simulink model "SatSim_ARES_prototype"  (R2022b)
settings: Solver=VariableStepAuto  StartTime=0.0  StopTime=100  RelTol=1e-3
values from neighbouring files (symbols this model uses):
  BC = m/A/Cd    (= 136.363636364)    [ARES.m]    (also in control_before_MPC.m = 122; reference_signal_291123.m = 121.212121212; validation.m)
  Cd = 2.2    [ARES.m]    (also in control_before_MPC.m; control_script_291123.m; reference_signal_291123.m; validation.m)
  CL = Cd*E    (= 0)    [ARES.m]    (also in control_before_MPC.m; control_script_291123.m; reference_signal_291123.m; validation.m)
  F107_avg = 90.85    [ARES.m]    (also in control_before_MPC.m; control_script_291123.m; reference_signal_291123.m; validation.m)
  F107_day = 86.0    (= 86)    [ARES.m]    (also in control_before_MPC.m; control_script_291123.m; reference_signal_291123.m; validation.m)
  jdate = jdate+ndays1    [ARES.m]    (also in control_before_MPC.m; control_script_291123.m; reference_signal_291123.m; validation.m)
  Kp = 1    [ARES.m]    (also in control_before_MPC.m; control_script_291123.m; reference_signal_291123.m; validation.m)
  mi = 398600.44    [ARES.m]    (also in control_before_MPC.m; control_script_291123.m; reference_signal_291123.m; validation.m)
  r_a = alt_0+Re    (= 6771.0088)    [ARES.m]    (also in control_before_MPC.m = 6571.0088; control_script_291123.m = 6571.0088; reference_signal_291123.m = 6571.0088; validation.m)
  Re = Re*1000    (= 6371008.8)    [ARES.m]    (also in control_before_MPC.m; control_script_291123.m; reference_signal_291123.m; trajectory_solver.m = 6378000)
  stop_h = 0    [ARES.m]    (also in control_before_MPC.m; control_script_291123.m; reference_signal_291123.m; validation.m)
libraries: simulink x2
settings Model: PauseTimes=0  Creator=zhanghanwen  LastModifiedBy=zhanghanwen

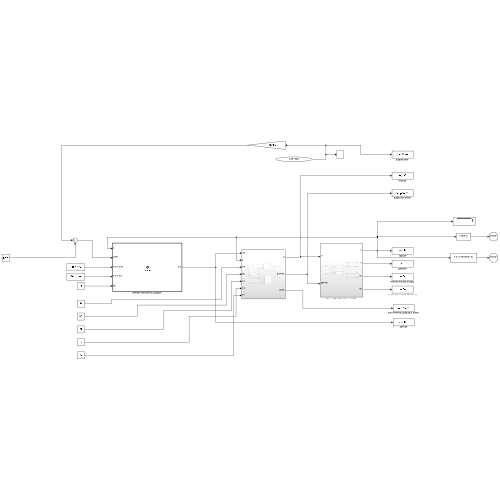
[thumbnail: Simulink's stored preview of the top-level diagram]
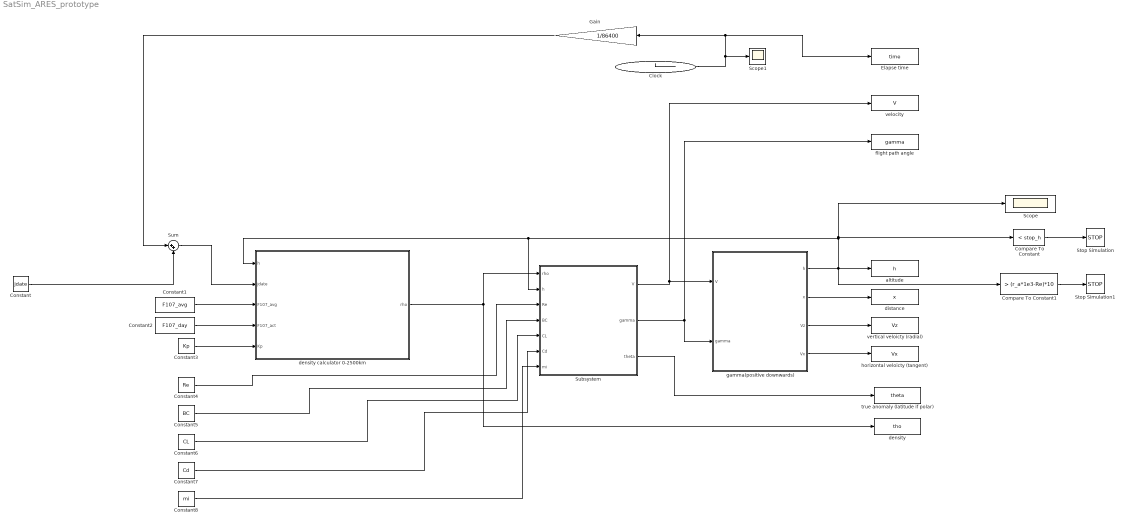
== system SatSim_ARES_prototype ==
  Clock : Clock
  Compare To Constant : simulink/Logic and Bit Operations/Compare To Constant  relop=<  const=stop_h  OutDataTypeStr=boolean
  Compare To Constant1 : simulink/Logic and Bit Operations/Compare To Constant  relop=>  const=(r_a*1e3-Re)*10  OutDataTypeStr=boolean
  Constant : Constant  Value=jdate
  Constant1 : Constant  Value=F107_avg
  Constant2 : Constant  Value=F107_day
  Constant3 : Constant  Value=Kp
  Constant4 : Constant  Value=Re
  Constant5 : Constant  Value=BC
  Constant6 : Constant  Value=CL
  Constant7 : Constant  Value=Cd
  Constant8 : Constant  Value=mi
  Elapse time : ToWorkspace  VariableName=time  SampleTime=-1
      settings: Save2DSignal=2-D array (concatenate along first dimension)
  Gain : Gain  Gain=1/86400
  Scope : Scope
  Scope1 : Scope
  Stop Simulation : Stop
  Stop Simulation1 : Stop
  Subsystem : Subsystem
  Sum : Sum  Inputs=|++
  altitude : ToWorkspace  VariableName=h  SampleTime=-1
      settings: Save2DSignal=2-D array (concatenate along first dimension)
  density : ToWorkspace  VariableName=tho  SampleTime=-1
      settings: Save2DSignal=2-D array (concatenate along first dimension)
  density calculator 0-2500km : MATLAB Function  TreatAsAtomicUnit=on
  distance : ToWorkspace  VariableName=x  SampleTime=-1
      settings: Save2DSignal=2-D array (concatenate along first dimension)
  flight path angle : ToWorkspace  VariableName=gamma  SampleTime=-1
      settings: Save2DSignal=2-D array (concatenate along first dimension)
  gamma(positive downwards) : Subsystem
  horizontal veloicty (tangent) : ToWorkspace  VariableName=Vx  SampleTime=-1
      settings: Save2DSignal=2-D array (concatenate along first dimension)
  true anomaly (latitude if polar) : ToWorkspace  VariableName=theta  SampleTime=-1
      settings: Save2DSignal=2-D array (concatenate along first dimension)
  velocity : ToWorkspace  VariableName=V  SampleTime=-1
      settings: Save2DSignal=2-D array (concatenate along first dimension)
  vertical veloicty (radial) : ToWorkspace  VariableName=Vz  SampleTime=-1
      settings: Save2DSignal=2-D array (concatenate along first dimension)
  wires:
  Constant1/1 -> density calculator 0-2500km/3(F107_avg)
  Constant3/1 -> density calculator 0-2500km/5(Kp)
  Constant2/1 -> density calculator 0-2500km/4(F107_act)
  Constant/1 -> Sum/2
  density calculator 0-2500km/1(rho) -> density/1, Subsystem/1(rho)
  Subsystem/1(V) -> velocity/1, gamma(positive downwards)/1(V)
  Subsystem/2(gamma) -> flight path angle/1, gamma(positive downwards)/2(gamma)
  gamma(positive downwards)/2(x) -> distance/1
  gamma(positive downwards)/3(Vz) -> vertical veloicty (radial)/1
  gamma(positive downwards)/4(Vx) -> horizontal veloicty (tangent)/1
  gamma(positive downwards)/1(h) -> Scope/1, Compare To Constant/1, density calculator 0-2500km/1(h), Subsystem/2(h), altitude/1, Compare To Constant1/1
  Compare To Constant1/1 -> Stop Simulation1/1
  Compare To Constant/1 -> Stop Simulation/1
  Subsystem/3(theta) -> true anomaly (latitude if polar)/1
  Gain/1 -> Sum/1
  Sum/1 -> density calculator 0-2500km/2(jdate)
  Constant6/1 -> Subsystem/5(CL)
  Constant5/1 -> Subsystem/4(BC)
  Constant7/1 -> Subsystem/6(Cd)
  Constant4/1 -> Subsystem/3(Re)
  Constant8/1 -> Subsystem/7(mi)
  Clock/1 -> Elapse time/1, Gain/1, Scope1/1

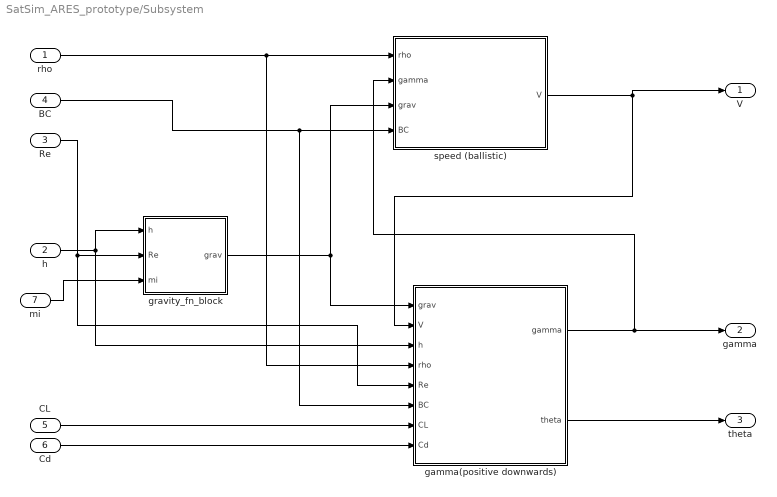
== system SatSim_ARES_prototype/Subsystem ==
  rho : Inport
  h : Inport  Port=2
  Re : Inport  Port=3
  BC : Inport  Port=4
  CL : Inport  Port=5
  Cd : Inport  Port=6
  mi : Inport  Port=7
  gamma(positive downwards) : Subsystem
  gravity_fn_block : MATLAB Function  TreatAsAtomicUnit=on
  speed (ballistic) : Subsystem
  V : Outport
  gamma : Outport  Port=2
  theta : Outport  Port=3
  wires:
  rho/1 -> gamma(positive downwards)/4(rho), speed (ballistic)/1(rho)
  gravity_fn_block/1(grav) -> speed (ballistic)/3(grav), gamma(positive downwards)/1(grav)
  h/1 -> gamma(positive downwards)/3(h), gravity_fn_block/1(h)
  gamma(positive downwards)/1(gamma) -> speed (ballistic)/2(gamma), gamma/1
  gamma(positive downwards)/2(theta) -> theta/1
  speed (ballistic)/1(V) -> V/1, gamma(positive downwards)/2(V)
  Re/1 -> gamma(positive downwards)/5(Re), gravity_fn_block/2(Re)
  BC/1 -> gamma(positive downwards)/6(BC), speed (ballistic)/4(BC)
  CL/1 -> gamma(positive downwards)/7(CL)
  Cd/1 -> gamma(positive downwards)/8(Cd)
  mi/1 -> gravity_fn_block/3(mi)

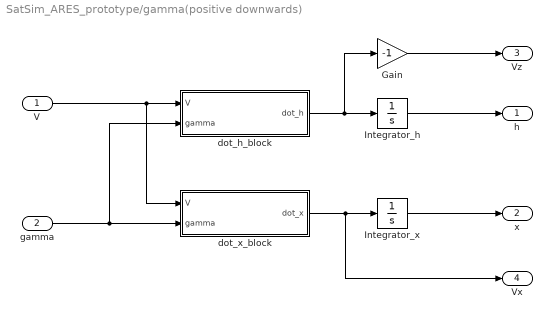
== system SatSim_ARES_prototype/gamma(positive downwards) ==
  V : Inport
  gamma : Inport  Port=2
  Gain : Gain  Gain=-1
  Integrator_h : Integrator
  Integrator_x : Integrator
  dot_h_block : MATLAB Function  TreatAsAtomicUnit=on
  dot_x_block : MATLAB Function  TreatAsAtomicUnit=on
  h : Outport
  x : Outport  Port=2
  Vz : Outport  Port=3
  Vx : Outport  Port=4
  wires:
  V/1 -> dot_x_block/1(V), dot_h_block/1(V)
  gamma/1 -> dot_x_block/2(gamma), dot_h_block/2(gamma)
  Integrator_h/1 -> h/1
  dot_h_block/1(dot_h) -> Gain/1, Integrator_h/1
  Integrator_x/1 -> x/1
  dot_x_block/1(dot_x) -> Vx/1, Integrator_x/1
  Gain/1 -> Vz/1

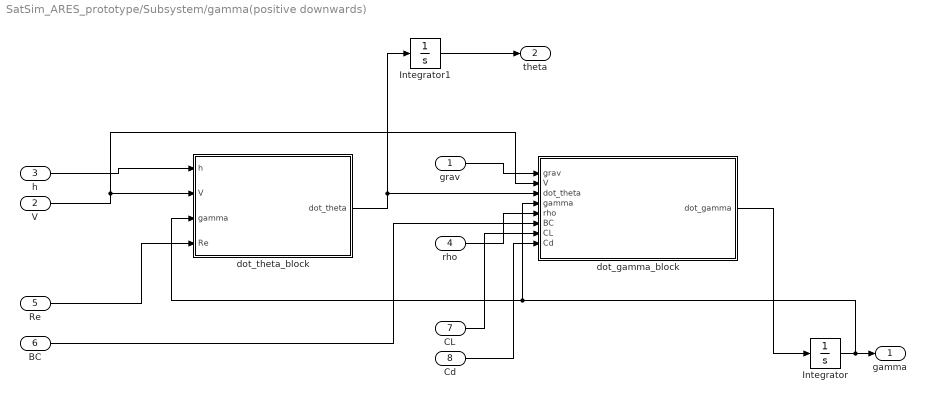
== system SatSim_ARES_prototype/Subsystem/gamma(positive downwards) ==
  grav : Inport
  V : Inport  Port=2
  h : Inport  Port=3
  rho : Inport  Port=4
  Re : Inport  Port=5
  BC : Inport  Port=6
  CL : Inport  Port=7
  Cd : Inport  Port=8
  Integrator : Integrator
  Integrator1 : Integrator
  dot_gamma_block : MATLAB Function  TreatAsAtomicUnit=on
  dot_theta_block : MATLAB Function  TreatAsAtomicUnit=on
  gamma : Outport
  theta : Outport  Port=2
  wires:
  grav/1 -> dot_gamma_block/1(grav)
  dot_gamma_block/1(dot_gamma) -> Integrator/1
  dot_theta_block/1(dot_theta) -> Integrator1/1, dot_gamma_block/3(dot_theta)
  rho/1 -> dot_gamma_block/5(rho)
  h/1 -> dot_theta_block/1(h)
  V/1 -> dot_gamma_block/2(V), dot_theta_block/2(V)
  Integrator1/1 -> theta/1
  Integrator/1 -> dot_theta_block/3(gamma), dot_gamma_block/4(gamma), gamma/1
  Re/1 -> dot_theta_block/4(Re)
  BC/1 -> dot_gamma_block/6(BC)
  CL/1 -> dot_gamma_block/7(CL)
  Cd/1 -> dot_gamma_block/8(Cd)

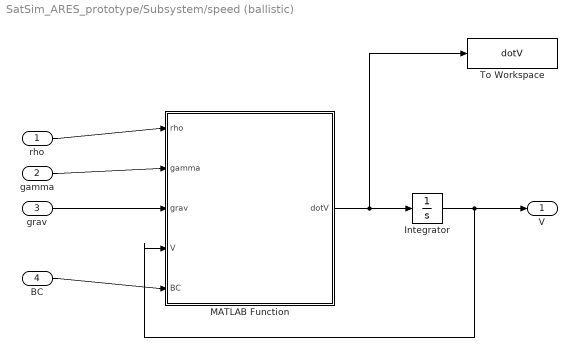
== system SatSim_ARES_prototype/Subsystem/speed (ballistic) ==
  rho : Inport
  gamma : Inport  Port=2
  grav : Inport  Port=3
  BC : Inport  Port=4
  Integrator : Integrator
  MATLAB Function : MATLAB Function  TreatAsAtomicUnit=on
  To Workspace : ToWorkspace  VariableName=dotV  SaveFormat=Timeseries  SampleTime=-1
  V : Outport
  wires:
  Integrator/1 -> MATLAB Function/4(V), V/1
  grav/1 -> MATLAB Function/3(grav)
  gamma/1 -> MATLAB Function/2(gamma)
  rho/1 -> MATLAB Function/1(rho)
  MATLAB Function/1(dotV) -> To Workspace/1, Integrator/1
  BC/1 -> MATLAB Function/5(BC)

== matlab function SatSim_ARES_prototype/Subsystem/gravity_fn_block ==
  data: h input; grav output; Re input; mi input
function grav = gravity(h,Re,mi)

grav = mi*1e9 / (Re+h)^2;
end

== matlab function SatSim_ARES_prototype/density calculator 0-2500km ==
  data: h input; jdate input; F107_avg input; rho output; F107_act input; Kp input
%This function combines Jacchia J71 and Exponential Atmosphere for %calculating density in the band [0;2500] km
%A transition function should be introduced to avoid discontinuities
function rho = unirho(h,jdate,F107_avg,F107_act,Kp) 
     h=h/1000; %conversion [m] to [km]
    rho=0;
    %from 0 to 100 km of altitude use Exponential Atmosphere
    if h<100 && h>=0
        rho=expAtm(h);
    end
    %from 100 to 2500 km of altitude use Jacchia J71
    if h>=100 && h<=2500 
       rho=J71_density_simulink(h,jdate,F107_avg,F107_act,Kp);
    end
    %A warning is printed if a negative altitude is predicted by %the simulation (due to Simulink discrete stopping criterion)
    if h<0
       fprintf('Warning: mismatched density, altitude: %3.2e km',h) 
       rho=1.225;
    end
end



%This function computes the density using Jacchia J71 model
%rho=J71_density_simulink(H,jdate,F107_avg,F107_act,Kp)
%input: height [90-2500 km], julian date, F10.7 3-monthly average, F10.7
%three hourly average, Kp planetary index
%output: density value
%Reference: Satellite Orbits, section 3.5.3
function rho=J71_density_simulink(H,jdate,F107_avg,F107_act,Kp)

    %% Exosperic Temperature 
    T_c = 379.0+3.24*F107_avg+1.3*(F107_act-F107_avg);
    % Geographic corrections
    % The actual exospheric temperature depends on the local hour angle
    % of the Sun with respect to the satellite.
    % It also depends, however, on the declination of the Sun and the
    % geographic latitude of the satellite.
    % The actual exospheric temperature T1 with the diurnal variations
    % included can be computed from a more compliated formula available
    % in the referenced book.
    % Geomagnetic corrections
    % using the three-hourly planetary geomagnetic index Kp for a time
    % 6.7 hours earlier than the time under consideration
    f = 0.5*(tanh(0.04*(H-350)+1));
    dT_infH = 28.0*Kp+0.03*exp(Kp);
    dT_infL = 14.0*Kp+0.02*exp(Kp);
    dT_gm = f*dT_infH+(1-f)*dT_infL;
    %transition function
    %H>350km
    %H<350km
    T_e = T_c+dT_gm;   %geomagnetic corrected exospheric temperature
    
    %% Standard Density 
    %Use bi-polynomial fit from Gill (1996)
    coeff=getCoeff(H,T_e); %coefficient matrix
    logRho=0;
    for i=0:5
        for j=0:4
            logRho = logRho + coeff(i+1,j+1)*((H/1000)^i)*((T_e/1000)^j);
        end 
    end

    %% Corrections 
    %Correction due to semi-annual density variation in thermosphere
    Phi=(jdate - 2400000.5 -36204)/365.2422; %number of tropical years since Jan1, 1958
    
    tauSA=Phi + 0.09544*((0.5+0.5*sin(2*pi*Phi+6.035))^1.65 - 0.5);
    fZ=(5.876e-7*H^2.331 + 0.06328)*exp(H*-2.868e-3);
    gt=0.02835 + 0.3817*(1+0.4671*sin(2*pi*tauSA+4.137))*sin(4*pi*tauSA+4.259);
    logRhoSA=fZ*gt;
    %Correction due to geomagnetic activities
     if H<350
            logRhoGM = (0.012*Kp + 1.2e-5*exp(Kp))*(1-f);%Transition function from temp calc
     else
        logRhoGM=0;
     end
    %Seasonal-latitude correction
    %logRhoSL=0.014*(Z-90).*exp(-0.0013*(Z-90).^2)*sin(1*pi*Phi -1.72)*sin(lat)^3/abs(sin(lat));
    logRho=logRho+logRhoGM+logRhoSA;
    rho=10^logRho;
end

%This function calculates density through an exponential model
%rho=expAtm(H)
%H is the geopotential height in km
%rho is the density in kg/m^3
%rho0,h0,SH are updated each 10 km (source: Wertz, 1978)
function rho=expAtm(H)
[rho0,h0,SH]=getSH(H);
rho=rho0*exp(-(H-h0)/SH);   %kg/m^3
end

function c=getCoeff(Z,T)
    %Retrieve coefficients for bi-polynomial fit taken from Tables 3.9 and 3.10
    %of Satellite Orbits. These numbers were entered manually and may include
    %some typing errors. This should be replaced by the process described in
    %E. Gill, "Smooth Bi-Polynomial Interpolation of Jacchia 1971 Atmospheric
    %Densities For Efficient Satellite Drag Computation," DLR-GSOC IB 96-1,
    %German Aerospace Center (DLR), 1996
    %This paper is unavailable at this time.
    if Z<90 || Z>2500
        error('Z must be in range 90km < Z < 2500km')
    end
    if T<500 || T>1900
        error('T must be in range 500K < T < 1900K')
    end
    if T<850
        if Z<1000
            if Z<500
                if Z<180
                    c=[-0.3520856e2  0.3912622e1 -0.8649259e2  0.1504119e3 -0.7109428e2 ...
                        0.1129210e4  0.1198158e4  0.8633794e3 -0.3577091e4 -0.1970558e4 ...
                       -0.1527475e5 -0.3558481e5  0.1899243e5  0.2508241e5 -0.1968253e5 ...
                        0.9302042e5  0.3646554e6 -0.3290364e6 -0.1209631e5 0.8438137e5...
                       -0.2734394e6 -0.1576097e7  0.1685831e7 -0.4282943e6 -0.1345593e6...
                        0.3149696e6  0.2487723e7 -0.2899124e7  0.1111904e7 0.3294095e4];
                else
                    c=[ 0.2311910e2  0.1355298e3 -0.8424310e3  0.1287331e4 -0.6181209e3...
                       -0.1057776e4  0.6087973e3  0.8690566e4 -0.1715922e5 0.9052671e4...
                        0.1177230e5 -0.3164132e5 -0.1076323e4  0.6302629e5 -0.4312459e5...
                       -0.5827663e5  0.2188167e6 -0.2422912e6  0.2461286e5 0.6044096e5...
                        0.1254589e6 -0.5434710e6  0.8123016e6 -0.4490438e6 0.5007458e5...
                       -0.9452922e5  0.4408026e6 -0.7379410e6  0.5095273e6 -0.1154192e6];
                end
            else
                c=[-0.1815722e4  0.9792972e4 -0.1831374e5  0.1385255e5 -0.3451234e4...
                    0.9851221e4 -0.5397525e5  0.9993169e5 -0.7259456e5 0.1622553e5...
                   -0.1822932e5  0.1002430e6 -0.1784481e6  0.1145178e6 -0.1641934e5...
                    0.1298113e5 -0.7113430e5  0.1106375e6 -0.3825777e5 -0.1666915e5...
                   -0.1533510e4  0.7815537e4  0.7037562e4 -0.4674636e5 0.3516946e5...
                   -0.1263680e4  0.7265792e4 -0.2092909e5  0.2936094e5 -0.1491676e5];
            end
        else
            c=[ 0.3548698e3 -0.2508685e4  0.6252742e4 -0.6755376e4  0.2675763e4...
               -0.5370852e3  0.4182586e4 -0.1151114e5  0.1338915e5 -0.5610580e4...
               -0.2349586e2 -0.8941841e3  0.4417927e4 -0.6732817e4  0.3312608e4...
                0.3407073e3 -0.1531588e4  0.2179045e4 -0.8841341e3 -0.1369769e3...
               -0.1698470e3  0.8985697e3 -0.1704797e4  0.1363098e4 -0.3812417e3...
                0.2494943e2 -0.1389618e3  0.2820058e3 -0.2472862e3  0.7896439e2];
        end
    else 
        if Z<1000
            if Z<500
                if Z<180
                     c=[-0.5335412e2  0.2900557e2 -0.2046439e2  0.7977149e1 -0.1335853e1...
                         0.1977533e4 -0.7091478e3  0.4398538e3 -0.1568720e3 0.2615466e2...
                         -0.2993620e5  0.5187286e4 -0.1989795e4  0.3643166e3 -0.5700669e2...
                         0.2112068e6 -0.4483029e4 -0.1349971e5  0.9510012e4 -0.1653725e4...
                         -0.7209722e6 -0.7684101e5  0.1256236e6 -0.6805699e5 0.1181257e5...
                         0.9625966e6  0.2123127e6 -0.2622793e6  0.1337130e6 -0.2329995e5];
                else
                    c=[ 0.4041761e2 -0.1305719e3  0.1466809e3 -0.7120296e2 0.1269605e2...
                       -0.8127720e3  0.2273565e4 -0.2577261e4  0.1259045e4 -0.2254978e3...
                        0.5130043e4 -0.1501308e5  0.1717142e5 -0.8441698e4 0.1518796e4...
                       -0.1600170e5  0.4770469e5 -0.5473492e5  0.2699668e5 -0.4870306e4...
                        0.2384718e5 -0.7199064e5  0.8284653e5 -0.4098358e5 0.7411926e4...
                       -0.1363104e5  0.4153499e5 -0.4793581e5  0.2377854e5 -0.4310233e4];
                end
            else
                c=[-0.4021335e2 -0.1326983e3  0.3778864e3 -0.2808660e3 0.6513531e2...
                    0.4255789e3  0.3528126e3 -0.2077888e4  0.1726543e4 -0.4191477e3...
                   -0.1821662e4  0.7905357e3  0.3934271e4 -0.3969334e4 0.1027991e4...
                    0.3070231e4 -0.2941540e4 -0.3276639e4  0.4420217e4 -0.1230778e4...
                   -0.2196848e4  0.2585118e4  0.1382776e4 -0.2533006e4 0.7451387e3...
                    0.5494959e3 -0.6604225e3 -0.3328077e3  0.6335703e3 -0.1879812e3];
            end
        else 
            c=[ 0.1281061e2 -0.3389179e3  0.6861935e3 -0.4667627e3  0.1029662e3...
                0.2024251e3  0.1668302e3 -0.1147876e4  0.9918940e3 -0.2430215e3...
               -0.5750743e3  0.8259823e3  0.2329832e3 -0.6503359e3  0.1997989e3...
                0.5106207e3 -0.1032012e4  0.4851874e3  0.8214097e2 -0.6527048e2...
               -0.1898953e3  0.4347501e3 -0.2986011e3  0.5423180e2  0.5039459e1...
                0.2569577e2 -0.6282710e2  0.4971077e2 -0.1404385e2  0.8450500e0];
        end
    end
end


%[rho0,h0,SH]=getSH(H) this function gives coefficient for an exponential
% atmosphere model
%works below 100 km
function [rho0,h0,SH]=getSH(H)
    %input data from table 8-4 of Fundamentals of Astrodynamics, D.A. Vallado
    h0=[0,25,30,40,50,60,70,80,90];
    rho0=[1.225,3.899e-2,1.774e-2,3.972e-3,1.057e-3,3.206e-4,8.770e-5,1.905e-5,3.396e-6];
    SH=[7.249,6.349,6.682,7.554,8.382,7.714,6.549,5.799,5.382];
    n=fix(H/10);
    if H>100 || H<0
        error('H must be in the range 0km < H < 100 km; current value H=%.2fkm\n',H) 
    end
    if H<30 
        n=2;
        if H<25 
            n=1;
        end 
    end
    if H==100
        n=9;
    end
    h0=h0(n);
    rho0=rho0(n);
    SH=SH(n);
end

== matlab function SatSim_ARES_prototype/Subsystem/speed (ballistic)/MATLAB Function ==
  data: rho input; dotV output; gamma input; grav input; V input; BC input
function dotV = dvdt(rho,gamma,grav,V,BC)
dotV = -0.5*rho*V^2/BC + grav*sin(gamma);
end

== matlab function SatSim_ARES_prototype/Subsystem/gamma(positive downwards)/dot_theta_block ==
  data: h input; dot_theta output; V input; gamma input; Re input
function dot_theta = dthetadt(h,V,gamma,Re)

dot_theta = V*cos(gamma)/(Re+h); 

end

== matlab function SatSim_ARES_prototype/Subsystem/gamma(positive downwards)/dot_gamma_block ==
  data: grav input; dot_gamma output; V input; dot_theta input; gamma input; rho input; BC input; CL input; Cd input
function dot_gamma = dgammadt(grav,V,dot_theta,gamma,rho,BC,CL,Cd)
dot_gamma = grav / V * cos(gamma) -dot_theta- 0.5 * rho/BC * CL / Cd*V; 
end

== matlab function SatSim_ARES_prototype/gamma(positive downwards)/dot_h_block ==
  data: V input; dot_h output; gamma input
function dot_h = dhdt(V,gamma)
dot_h = -V*sin(gamma);
end

== matlab function SatSim_ARES_prototype/gamma(positive downwards)/dot_x_block ==
  data: V input; dot_x output; gamma input
function dot_x = dxdt(V,gamma)
dot_x = -V*cos(gamma);
end
